simulink model "asynchronous_motor_capacitor_reactive_power"  (R2017b)
settings: Solver=VariableStepAuto  StartTime=0.0  StopTime=20  MaxStep=1e-4  RelTol=1e-3
undefined symbols (not defined in the file): magnitude
libraries: powerlib x6, sdolib x1, powerlib_meascontrol x1
settings Model: Creator=Damla  LastModifiedBy=dagac

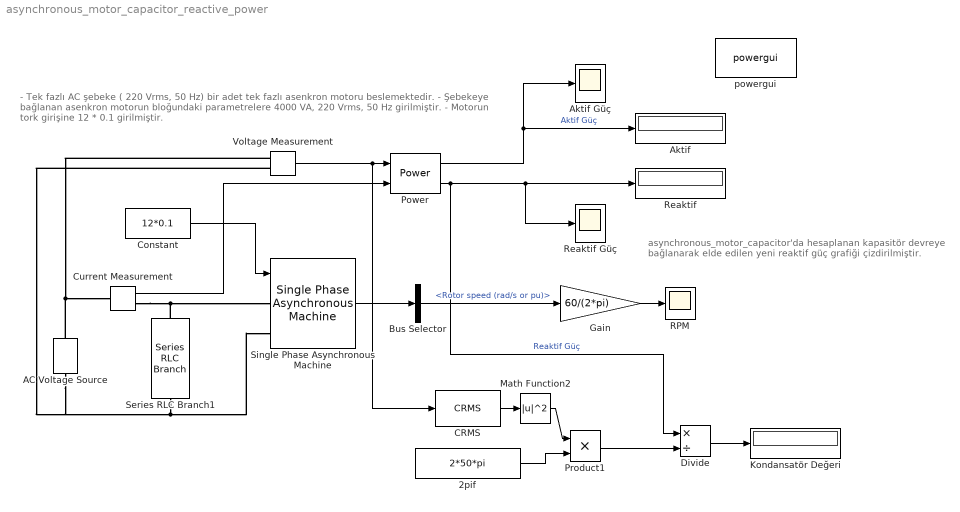
== system asynchronous_motor_capacitor_reactive_power ==
  note: asynchronous_motor_capacitor'da hesaplanan kapasitör
      | devreye bağlanarak elde edilen yeni reaktif güç grafiği çizdirilmiştir.
  note: - Tek fazlı AC şebeke ( 220 Vrms, 50 Hz) bir adet tek fazlı asenkron motoru beslemektedir.
      | - Şebekeye bağlanan asenkron motorun bloğundaki parametrelere 4000 VA, 220 Vrms, 50 Hz girilmiştir.
      | - Motorun tork girişine 12 * 0.1 girilmiştir.
  "2pif " : Constant  Value=2*50*pi
  AC Voltage Source : powerlib/Electrical Sources/AC Voltage Source  Amplitude=311.12  Phase=0  Frequency=50  SampleTime=0  Measurements=None  BusType=swing  Pref=10e3  Qref=0  Qmin=-inf  Qmax=+inf
  Aktif : Display
  Aktif Güç : Scope
  Bus Selector : BusSelector  OutputSignals=Mechanical.Rotor speed (rad/s or pu)
  CRMS : sdolib/RMS Blocks/CRMS
      settings: SourceProductName=Simulink Design Optimization  SourceProductBaseCode=SO
  Constant : Constant  Value=12*0.1
  Current Measurement : powerlib/Measurements/Current Measurement  PhasorSimulation=off  OutputType=Complex  PSBequivalent=0
  Divide : Product  Inputs=*/
  Gain : Gain  Gain=60/(2*pi)
  Kondansatör Değeri : Display
  Math Function2 : Math  Operator=magnitude^2  SaturateOnIntegerOverflow=on
  Power : powerlib_meascontrol/Measurements/Power  Freq=50  Vinit=[1, 0]  Iinit=[1, 0]  Ts=0
      settings: SourceProductName=Simscape Power Systems
  Product1 : Product
  RPM : Scope
  Reaktif : Display
  Reaktif Güç : Scope
  Series RLC Branch1 : powerlib/Elements/Series RLC Branch  LConnTagsString=__new0  RConnTagsString=__new0  BranchType=RC  Resistance=0.1  Inductance=0.01  SetiL0=off  InitialCurrent=0  Capacitance=9.918e-05  Setx0=off  InitialVoltage=0  Measurements=None
  Single Phase Asynchronous Machine : powerlib/Machines/Single Phase Asynchronous Machine  MechanicalLoad=Torque Tm  UNITS=SI  MachineType=Split Phase  MeasurementBus=off  NominalParameters="[ 4000  220  50]"  MainWindingStator="[2.02  7.4e-3]"  MainWindingRotor="[4.12  5.6e-3]"  MutualInductance=0.1772  AuxiliaryWinding="[7.14  8.5e-3]"  Mechanical="[0.0146  0  2 1.18]"  CapacitorStart="[2  254.7e-6]"  CapacitorRun="[18  21.1e-6]"  DisconnectionSpeed=75  InitialSpeed=0  DataType=SI  TsPowergui=0  TsBlock=-1
      settings: SourceProductName=Simscape Power Systems  SourceProductBaseCode=PS
  Voltage Measurement : powerlib/Measurements/Voltage Measurement  PhasorSimulation=off  OutputType=Complex  PSBequivalent=0
  powergui : powerlib/powergui  Priority=1  SimulationMode=Continuous  SampleTime=50e-6  frequency=60  Iterations=50  frequencyindice=50  Pbase=100e6  ErrMax=1e-4  UnitsV=kV  UnitsW=MW  buscounter=0  FunctionMessages=off  echomessages=off  EnableUseOfTLC=off  CurrentSourceSwitches=off  DisableSnubberDevices=off  DisableRonSwitches=off  DisableVfSwitches=off  DisplayEquations=off  SolverType=Tustin/Backward Euler (TBE)  Interpol=off  ExternalGateDelay=off  methode=off  Ts=100  x0status=blocks  SPID=on  SwTol=0  HookPort=off  RestoreLinks=warning  ResistiveCurrentMeasurement=off  Frange=[0:2:500]  Ylog=off  Xlog=on  ShowGrid=off  save=off  variable=ZData  structure=0  ZoomFFT=off  StartTime=0.0  cycles=1  DisplayStyle=1  fundamental=60  FreqAxis=off  MaxFrequency=1000  frequencyindicesteady=1  RmsSteady=1  display=off
  wires:
  Constant/1 -> Single Phase Asynchronous Machine/1
  Gain/1 -> RPM/1
  Current Measurement/1 -> Power/2
  Single Phase Asynchronous Machine/1 -> Bus Selector/1
  Bus Selector/1 -> Gain/1  "<Rotor speed (rad/s or pu)>"
  Power/1 -> Aktif Güç/1, Aktif/1  "Aktif Güç"
  Voltage Measurement/1 -> CRMS/1, Power/1
  Power/2 -> Divide/1, Reaktif Güç/1, Reaktif/1  "Reaktif Güç"
  CRMS/1 -> Math Function2/1
  Divide/1 -> Kondansatör Değeri/1
  Math Function2/1 -> Product1/1
  Product1/1 -> Divide/2
  "2pif "/1 -> Product1/2
  connections:
  AC Voltage Source/LConn1 -- Voltage Measurement/LConn2 -- Series RLC Branch1/RConn1 -- Single Phase Asynchronous Machine/LConn2
  AC Voltage Source/RConn1 -- Voltage Measurement/LConn1 -- Current Measurement/LConn1
  Current Measurement/RConn1 -- Series RLC Branch1/LConn1 -- Single Phase Asynchronous Machine/LConn1
